simulink model "Active_Suspension_Control_Simulink_TEST"  (R2023b)
settings: Solver=FixedStepAuto  StartTime=0.0  StopTime=10  FixedStep=0.001  MaxStep=1e-3  RelTol=1e-3
values from neighbouring files (symbols this model uses):
  a = [1 20 3486.66666667 10555.5555556 168888.888889]    [Fuzzy_Workspace.mat]    (also in quarter_car_model.m = 0.8)
  b = [0 0 0.00333333333333 10555.6111112 168900.333335]    [Fuzzy_Workspace.mat]
  c_car = 1000    [Active_Suspension_Control.m]    (also in Fuzzy_Workspace.mat)
  k_car = 16000    [Active_Suspension_Control.m]    (also in Fuzzy_Workspace.mat)
  k_wheel = 190000    [Active_Suspension_Control.m]    (also in Fuzzy_Workspace.mat)
  m_car = 300    [Active_Suspension_Control.m]    (also in Fuzzy_Workspace.mat)
  m_wheel = 60    [Active_Suspension_Control.m]    (also in Fuzzy_Workspace.mat)
libraries: slpidlib x2, fuzblock x1, simulink x1
settings Model: Creator=hkurt  LastModifiedBy=hkurt
settings SolverCC: ZeroCrossControl=DisableAll  EnableFixedStepZeroCrossing=on

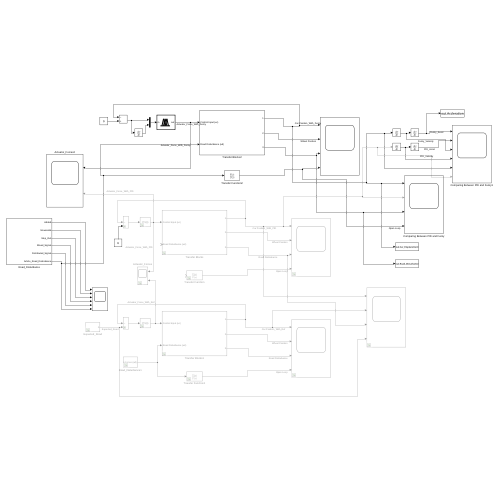
[thumbnail: Simulink's stored preview of the top-level diagram]
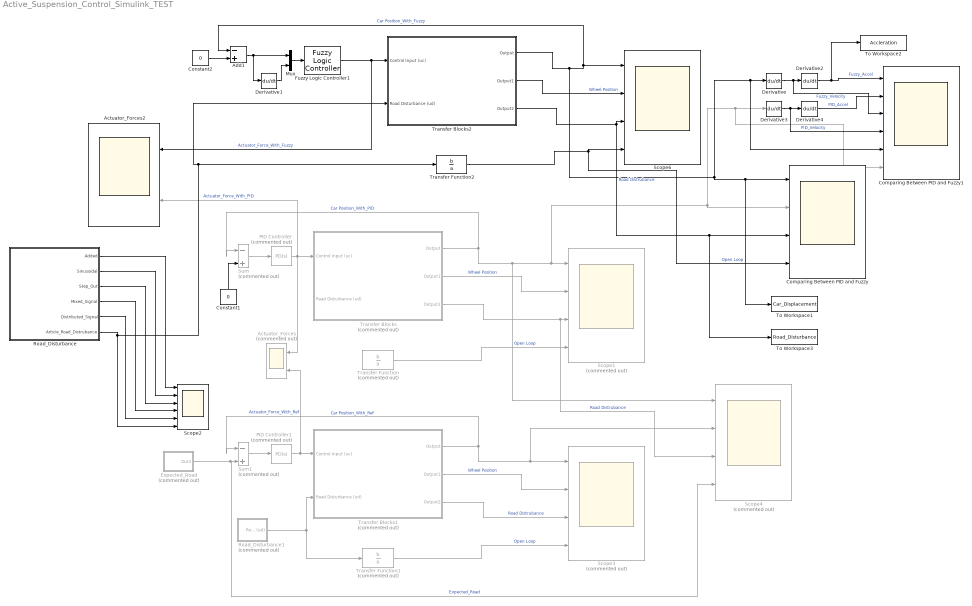
== system Active_Suspension_Control_Simulink_TEST ==
  Actuator_Forces : Scope  Commented=on  NumInputPorts=2
  Actuator_Forces2 : Scope  NumInputPorts=2
  Add1 : Sum  Inputs=-+
  Comparing Between PID and Fuzzy : Scope  NumInputPorts=4
  Comparing Between PID and Fuzzy1 : Scope  NumInputPorts=6
  Constant1 : Constant  Value=0
  Constant2 : Constant  Value=0
  Derivative{,1..4} (5 alike) : Derivative
  Expected_Road : Subsystem  Commented=on
  Fuzzy Logic Controller1 : fuzblock/Fuzzy Logic  Controller  FIS=my_fuzzy_8  OutputSampleNumber=101  DataType=double  FuzzifiedInputs=off  RuleFiringStrengths=off  RuleOutputs=off  AggregatedOutputs=off  SimulateUsing=Interpreted execution  OutOfRangeInputValueMessage=warning  NoRuleFiredMessage=warning  EmptyOutputFuzzySetMessage=warning
  Mux : Mux  Inputs=2
  PID Controller : slpidlib/PID Controller  Commented=on  Controller=PD  Form=Parallel  TimeDomain=Continuous-time  UseExternalTs=off  SampleTime=-1  IntegratorMethod=Forward Euler  FilterMethod=Forward Euler  ControllerParametersSource=internal  P=0.01  I=1000  UseKiTs=off  D=10000  N=100  UseFilter=on  TunerSelectOption=Transfer Function Based (PID Tuner App)  InitialConditionSource=internal  InitialConditionForIntegrator=0  InitialConditionForFilter=0  DifferentiatorICPrevScaledInput=0  ExternalReset=none  TrackingMode=off  Kt=1  LimitOutput=off  SatLimitsSource=internal  UpperSaturationLimit=2000  LowerSaturationLimit=-2000  LinearizeAsGain=on  AntiWindupMode=none  Kb=1  LimitIntegrator=off  UpperIntegratorSaturationLimit=inf  LowerIntegratorSaturationLimit=-inf  POutMin=[]  POutMax=[]  IOutMin=[]  IOutMax=[]  DOutMin=[]  DOutMax=[]  NOutMin=[]  NOutMax=[]  SumOutMin=[]  SumOutMax=[]  SaturationOutMin=[]  SaturationOutMax=[]  PParamMin=[]  PParamMax=[]  IParamMin=[]  IParamMax=[]  DParamMin=[]  DParamMax=[]  NParamMin=[]  NParamMax=[]  KbParamMin=[]  KbParamMax=[]  KtParamMin=[]  KtParamMax=[]  KbOutMin=[]  KbOutMax=[]  KtOutMin=[]  KtOutMax=[]  IntegratorOutMin=[]  IntegratorOutMax=[]  FilterOutMin=[]  FilterOutMax=[]  SumI1OutMin=[]  SumI1OutMax=[]  SumI2OutMin=[]  SumI2OutMax=[]  SumI3OutMin=[]  SumI3OutMax=[]  SumI4OutMin=[]  SumI4OutMax=[]  SumDOutMin=[]  SumDOutMax=[]  DifferentiatorOutMin=[]  DifferentiatorOutMax=[]  FilterDiffOutCoefMin=[]  FilterDiffOutCoefMax=[]  ReciprocalOutMin=[]  ReciprocalOutMax=[]  SumDenOutMin=[]  SumDenOutMax=[]  SumNumOutMin=[]  SumNumOutMax=[]  DivideOutMin=[]  DivideOutMax=[]  UdiffTsProdOutMin=[]  UdiffTsProdOutMax=[]  NTsProdOutMin=[]  NTsProdOutMax=[]  UintegralTsProdOutMin=[]  UintegralTsProdOutMax=[]  UngainTsProdOutMin=[]  UngainTsProdOutMax=[]  ClampingZeroOutDataTypeStr=Inherit: Inherit via back propagation  ClampingZeroOutMin=[]  ClampingZeroOutMax=[]  FilterDenConstantOutDataTypeStr=Inherit: Inherit via back propagation  FilterDenConstantOutMin=[]  FilterDenConstantOutMax=[]  PCopyOutDataTypeStr=Inherit: Inherit via back propagation  PCopyOutMin=[]  PCopyOutMax=[]  NCopyOutDataTypeStr=Inherit: Inherit via back propagation  NCopyOutMin=[]  NCopyOutMax=[]  IntegratorContinuousStateAttributes=''  IntegratorStateMustResolveToSignalObject=off  IntegratorRTWStateStorageClass=Auto  FilterContinuousStateAttributes=''  FilterStateMustResolveToSignalObject=off  FilterRTWStateStorageClass=Auto  ParallelPVariant=InternalParameters  IdealPVariant=Disabled  IVariant=Disabled  DVariant=InternalParameters  IntegratorVariant=Disabled  SatVariant=Disabled  AWVariant=Disabled  PCopyVariant=Disabled  TRVariant=Disabled  FdbkBlocksVariant=Forward  IdealPFdbkVariant=Disabled  SatFdbkVariant=Disabled  DerivativeFilterVariant=ContFilter  NVariant=InternalParameters  NCopyVariant=Disabled  FilterICVariant=InternalICsFilter  IntegratorICVariant=Disabled  ExternalResetVariant=Disabled  TRSumVariant=Passthrough  SumFdbkVariant=Disabled  SumVariant=Sum_PD  TsampFilterVariant=InternalTs  TsampNgainVariant=Passthrough  TsampIntegralVariant=Disabled_SignalSpec  ExternalSaturationOutDataTypeStr=Inherit: Same as second input
  PID Controller1 : slpidlib/PID Controller  Commented=on  Controller=PD  Form=Parallel  TimeDomain=Continuous-time  UseExternalTs=off  SampleTime=-1  IntegratorMethod=Forward Euler  FilterMethod=Forward Euler  ControllerParametersSource=internal  P=0.01  I=1000  UseKiTs=off  D=10000  N=100  UseFilter=on  TunerSelectOption=Transfer Function Based (PID Tuner App)  InitialConditionSource=internal  InitialConditionForIntegrator=0  InitialConditionForFilter=0  DifferentiatorICPrevScaledInput=0  ExternalReset=none  TrackingMode=off  Kt=1  LimitOutput=off  SatLimitsSource=internal  UpperSaturationLimit=2000  LowerSaturationLimit=-2000  LinearizeAsGain=on  AntiWindupMode=none  Kb=1  LimitIntegrator=off  UpperIntegratorSaturationLimit=inf  LowerIntegratorSaturationLimit=-inf  POutMin=[]  POutMax=[]  IOutMin=[]  IOutMax=[]  DOutMin=[]  DOutMax=[]  NOutMin=[]  NOutMax=[]  SumOutMin=[]  SumOutMax=[]  SaturationOutMin=[]  SaturationOutMax=[]  PParamMin=[]  PParamMax=[]  IParamMin=[]  IParamMax=[]  DParamMin=[]  DParamMax=[]  NParamMin=[]  NParamMax=[]  KbParamMin=[]  KbParamMax=[]  KtParamMin=[]  KtParamMax=[]  KbOutMin=[]  KbOutMax=[]  KtOutMin=[]  KtOutMax=[]  IntegratorOutMin=[]  IntegratorOutMax=[]  FilterOutMin=[]  FilterOutMax=[]  SumI1OutMin=[]  SumI1OutMax=[]  SumI2OutMin=[]  SumI2OutMax=[]  SumI3OutMin=[]  SumI3OutMax=[]  SumI4OutMin=[]  SumI4OutMax=[]  SumDOutMin=[]  SumDOutMax=[]  DifferentiatorOutMin=[]  DifferentiatorOutMax=[]  FilterDiffOutCoefMin=[]  FilterDiffOutCoefMax=[]  ReciprocalOutMin=[]  ReciprocalOutMax=[]  SumDenOutMin=[]  SumDenOutMax=[]  SumNumOutMin=[]  SumNumOutMax=[]  DivideOutMin=[]  DivideOutMax=[]  UdiffTsProdOutMin=[]  UdiffTsProdOutMax=[]  NTsProdOutMin=[]  NTsProdOutMax=[]  UintegralTsProdOutMin=[]  UintegralTsProdOutMax=[]  UngainTsProdOutMin=[]  UngainTsProdOutMax=[]  ClampingZeroOutDataTypeStr=Inherit: Inherit via back propagation  ClampingZeroOutMin=[]  ClampingZeroOutMax=[]  FilterDenConstantOutDataTypeStr=Inherit: Inherit via back propagation  FilterDenConstantOutMin=[]  FilterDenConstantOutMax=[]  PCopyOutDataTypeStr=Inherit: Inherit via back propagation  PCopyOutMin=[]  PCopyOutMax=[]  NCopyOutDataTypeStr=Inherit: Inherit via back propagation  NCopyOutMin=[]  NCopyOutMax=[]  IntegratorContinuousStateAttributes=''  IntegratorStateMustResolveToSignalObject=off  IntegratorRTWStateStorageClass=Auto  FilterContinuousStateAttributes=''  FilterStateMustResolveToSignalObject=off  FilterRTWStateStorageClass=Auto  ParallelPVariant=InternalParameters  IdealPVariant=Disabled  IVariant=Disabled  DVariant=InternalParameters  IntegratorVariant=Disabled  SatVariant=Disabled  AWVariant=Disabled  PCopyVariant=Disabled  TRVariant=Disabled  FdbkBlocksVariant=Forward  IdealPFdbkVariant=Disabled  SatFdbkVariant=Disabled  DerivativeFilterVariant=ContFilter  NVariant=InternalParameters  NCopyVariant=Disabled  FilterICVariant=InternalICsFilter  IntegratorICVariant=Disabled  ExternalResetVariant=Disabled  TRSumVariant=Passthrough  SumFdbkVariant=Disabled  SumVariant=Sum_PD  TsampFilterVariant=InternalTs  TsampNgainVariant=Passthrough  TsampIntegralVariant=Disabled_SignalSpec  ExternalSaturationOutDataTypeStr=Inherit: Same as second input
  Road_Disturbance : Subsystem
  Road_Disturbance1 : Subsystem  Commented=on
  Scope1 : Scope  Commented=on  NumInputPorts=4
  Scope2 : Scope  NumInputPorts=6
  Scope3 : Scope  Commented=on  NumInputPorts=4
  Scope4 : Scope  Commented=on  NumInputPorts=4
  Scope6 : Scope  NumInputPorts=4
  Sum : Sum  Commented=on  Inputs=|-+
  Sum1 : Sum  Commented=on  Inputs=|-+
  To Workspace1 : ToWorkspace  VariableName=Car_Displacement  SaveFormat=Timeseries  SampleTime=-1
  To Workspace2 : ToWorkspace  VariableName=Accleration  SaveFormat=Timeseries  SampleTime=-1
  To Workspace3 : ToWorkspace  VariableName=Road_Disturbance  SaveFormat=Timeseries  SampleTime=-1
  Transfer Blocks : Subsystem  Commented=on
  Transfer Blocks1 : Subsystem  Commented=on
  Transfer Blocks2 : Subsystem
  Transfer Function : TransferFcn  Commented=on  Numerator=b  Denominator=a
  Transfer Function1 : TransferFcn  Commented=on  Numerator=b  Denominator=a
  Transfer Function2 : TransferFcn  Numerator=b  Denominator=a
  wires:
  Transfer Blocks/2(Output1) -> Scope1/2  "Wheel Position"
  Transfer Blocks/3(Output2) -> Scope4/3, Scope1/3  "Road Distrubance"
  Transfer Blocks/1(Output) -> Sum/1, Scope4/1, Comparing Between PID and Fuzzy1/6, Derivative3/1, Comparing Between PID and Fuzzy/2, Scope1/1  "Car Position_With_PID"
  Transfer Function/1 -> Scope1/4  "Open Loop"
  Sum/1 -> PID Controller/1
  PID Controller/1 -> Actuator_Forces2/2, Actuator_Forces/1, Transfer Blocks/1(Control Input (uc))  "Actuator_Force_With_PID"
  Transfer Function1/1 -> Scope3/4  "Open Loop"
  Transfer Blocks1/3(Output2) -> Scope3/3  "Road Distrubance"
  Sum1/1 -> PID Controller1/1
  Transfer Blocks1/1(Output) -> Sum1/1, Scope4/2, Scope3/1  "Car Position_With_Ref"
  Road_Disturbance1/1(Road Disturbance (ud)) -> Transfer Blocks1/2(Road Disturbance (ud)), Transfer Function1/1
  PID Controller1/1 -> Actuator_Forces/2, Transfer Blocks1/1(Control Input (uc))  "Actuator_Force_With_Ref"
  Transfer Blocks1/2(Output1) -> Scope3/2  "Wheel Position"
  Expected_Road/1(Out1) -> Scope4/4, Sum1/2  "Expected_Road"
  Constant1/1 -> Sum/2
  Transfer Function2/1 -> Comparing Between PID and Fuzzy/4, Scope6/4  "Open Loop"
  Transfer Blocks2/3(Output2) -> To Workspace3/1, Comparing Between PID and Fuzzy/3, Scope6/3  "Road Distrubance"
  Transfer Blocks2/2(Output1) -> Scope6/2  "Wheel Position"
  Transfer Blocks2/1(Output) -> Comparing Between PID and Fuzzy1/5, Derivative/1, To Workspace1/1, Comparing Between PID and Fuzzy/1, Add1/1, Scope6/1  "Car Position_With_Fuzzy"
  Add1/1 -> Derivative1/1, Mux/1
  Mux/1 -> Fuzzy Logic Controller1/1
  Derivative1/1 -> Mux/2
  Constant2/1 -> Add1/2
  Fuzzy Logic Controller1/1 -> Transfer Blocks2/1(Control Input (uc)), Actuator_Forces2/1  "Actuator_Force_With_Fuzzy"
  Derivative/1 -> Comparing Between PID and Fuzzy1/3, Derivative2/1  "Fuzzy_Velocity"
  Derivative3/1 -> Comparing Between PID and Fuzzy1/4, Derivative4/1  "PID_Velocity"
  Derivative4/1 -> Comparing Between PID and Fuzzy1/2  "PID_Accel"
  Derivative2/1 -> To Workspace2/1, Comparing Between PID and Fuzzy1/1  "Fuzzy_Accel"
  Road_Disturbance/1(Added) -> Scope2/1
  Road_Disturbance/2(Sinusoidal) -> Scope2/2
  Road_Disturbance/3(Step_Out) -> Scope2/3
  Road_Disturbance/4(Mixed_Signal) -> Scope2/4
  Road_Disturbance/5(Distributed_Signal) -> Scope2/5
  Road_Disturbance/6(Article_Road_Distrubance) -> Scope2/6, Transfer Blocks2/2(Road Disturbance (ud)), Transfer Function2/1

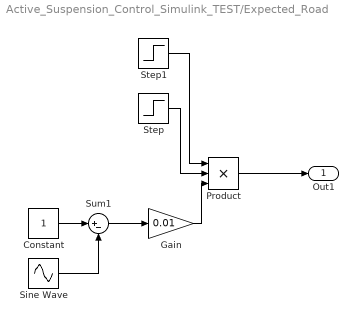
== system Active_Suspension_Control_Simulink_TEST/Expected_Road ==
  Constant : Constant
  Gain : Gain  Gain=0.01
  Product : Product  Inputs=3
  Sine Wave : Sin  Frequency=0.5*pi  Phase=pi/4  SampleTime=0
  Step : Step  Time=4.5  Before=1  After=0  SampleTime=0
  Step1 : Step  Time=0.5  SampleTime=0
  Sum1 : Sum  Inputs=|+-
  Out1 : Outport
  wires:
  Sine Wave/1 -> Sum1/2
  Sum1/1 -> Gain/1
  Gain/1 -> Product/3
  Step/1 -> Product/2
  Constant/1 -> Sum1/1
  Product/1 -> Out1/1
  Step1/1 -> Product/1

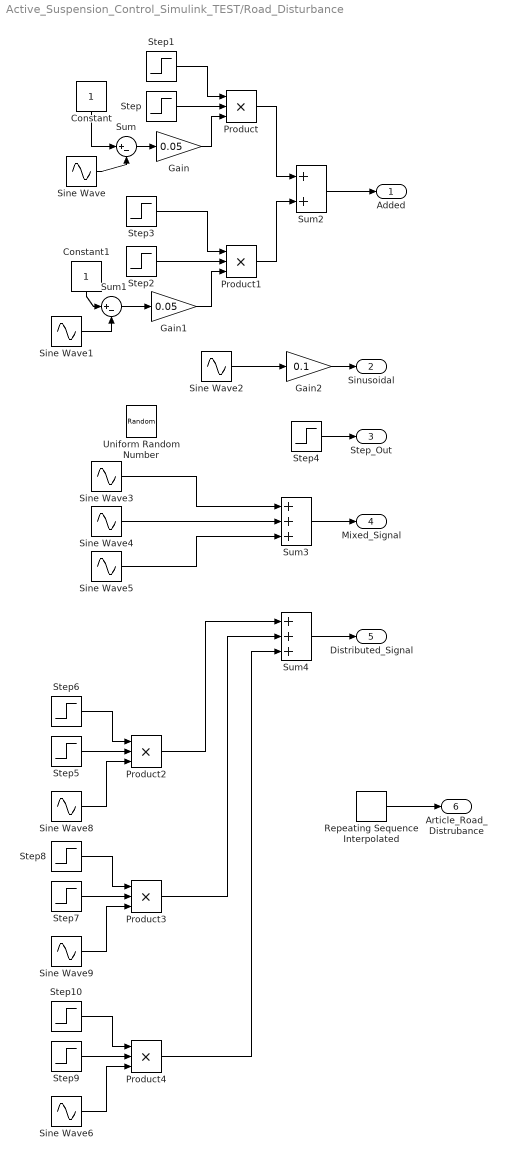
== system Active_Suspension_Control_Simulink_TEST/Road_Disturbance ==
  Constant : Constant
  Constant1 : Constant
  Gain : Gain  Gain=0.05
  Gain1 : Gain  Gain=0.05
  Gain2 : Gain  Gain=0.1
  Product{,1..4} (5 alike) : Product  Inputs=3
  Repeating Sequence Interpolated : simulink/Sources/Repeating Sequence Interpolated  OutValues=[0.0 -0.005 -0.012 -0.011 -0.015 0.012 0.009 0.028 0.024 0.020 0.026 0.028 0.020 -0.01 -0.012 -0.015 0.02 0.028 -0.018 0.02 0.015 0.012 -0.005 -0.013 0.007 0.0].'  TimeValues=[0 0.4 0.8 1.2 1.6 2.0 2.4 2.8 3.2 3.6 4.0 4.4 4.8 5.2 5.6 6.0 6.4 6.8 7.2 7.6 8.0 8.4 8.8 9.2 9.6 10.0].'  LookUpMeth=Interpolation-Use End Values  tsamp=0.01  OutMin=[]  OutMax=[]  OutDataTypeStr=double  OutputDataTypeScalingMode=double  OutDataType=fixdt(0,8)  OutScaling=2^-10
  Sine Wave : Sin  Frequency=2*pi  Phase=pi*3/2  SampleTime=0
  Sine Wave1 : Sin  Frequency=2*pi  Phase=pi*3/2  SampleTime=0
  Sine Wave2 : Sin  Frequency=2*pi  Phase=pi  SampleTime=0
  Sine Wave3 : Sin  Amplitude=0.01  Frequency=15*pi  SampleTime=0
  Sine Wave4 : Sin  Amplitude=0.02  Frequency=10*pi  Phase=pi/2  SampleTime=0
  Sine Wave5 : Sin  Amplitude=0.03  Frequency=pi  SampleTime=0
  Sine Wave6 : Sin  Amplitude=0.08  Frequency=pi  Phase=pi*3/2  SampleTime=0
  Sine Wave8 : Sin  Amplitude=0.1  Frequency=pi  Phase=pi*3/2  SampleTime=0
  Sine Wave9 : Sin  Amplitude=0.05  Frequency=pi  Phase=pi*3/2  SampleTime=0
  Step : Step  Time=1.5  Before=1  After=0  SampleTime=0
  Step1 : Step  Time=0.5  SampleTime=0
  Step10 : Step  Time=8.5  SampleTime=0
  Step2 : Step  Time=3.5  Before=1  After=0  SampleTime=0
  Step3 : Step  Time=2.5  SampleTime=0
  Step4 : Step  Time=2  After=0.015  SampleTime=0
  Step5 : Step  Time=1.5  Before=1  After=0  SampleTime=0
  Step6 : Step  Time=0.5  SampleTime=0
  Step7 : Step  Time=5.5  Before=1  After=0  SampleTime=0
  Step8 : Step  Time=4.5  SampleTime=0
  Step9 : Step  Time=9.5  Before=1  After=0  SampleTime=0
  Sum : Sum  Inputs=|+-
  Sum1 : Sum  Inputs=|+-
  Sum2 : Sum
  Sum3 : Sum  Inputs=+++
  Sum4 : Sum  Inputs=+++
  Uniform Random Number : UniformRandomNumber  Minimum=-0.05  Maximum=0.05  SampleTime=0.1
  Added : Outport
  Sinusoidal : Outport  Port=2
  Step_Out : Outport  Port=3
  Mixed_Signal : Outport  Port=4
  Distributed_Signal : Outport  Port=5
  Article_Road_Distrubance : Outport  Port=6
  wires:
  Constant/1 -> Sum/1
  Step/1 -> Product/2
  Sum/1 -> Gain/1
  Gain/1 -> Product/3
  Sine Wave/1 -> Sum/2
  Step1/1 -> Product/1
  Gain1/1 -> Product1/3
  Step2/1 -> Product1/2
  Step3/1 -> Product1/1
  Product1/1 -> Sum2/2
  Product/1 -> Sum2/1
  Constant1/1 -> Sum1/1
  Sine Wave1/1 -> Sum1/2
  Sum1/1 -> Gain1/1
  Sine Wave2/1 -> Gain2/1
  Sum2/1 -> Added/1
  Gain2/1 -> Sinusoidal/1
  Step4/1 -> Step_Out/1
  Sum3/1 -> Mixed_Signal/1
  Sine Wave3/1 -> Sum3/1
  Sine Wave4/1 -> Sum3/2
  Sine Wave5/1 -> Sum3/3
  Step6/1 -> Product2/1
  Product2/1 -> Sum4/1
  Step5/1 -> Product2/2
  Sine Wave8/1 -> Product2/3
  Sum4/1 -> Distributed_Signal/1
  Step8/1 -> Product3/1
  Step7/1 -> Product3/2
  Sine Wave9/1 -> Product3/3
  Product3/1 -> Sum4/2
  Step10/1 -> Product4/1
  Step9/1 -> Product4/2
  Sine Wave6/1 -> Product4/3
  Product4/1 -> Sum4/3
  Repeating Sequence Interpolated/1 -> Article_Road_Distrubance/1

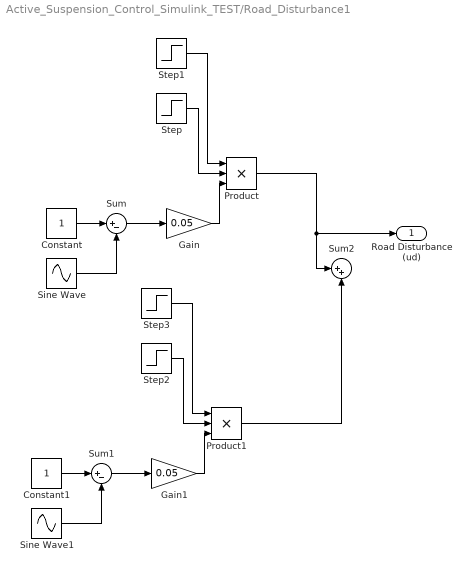
== system Active_Suspension_Control_Simulink_TEST/Road_Disturbance1 ==
  Constant : Constant
  Constant1 : Constant
  Gain : Gain  Gain=0.05
  Gain1 : Gain  Gain=0.05
  Product : Product  Inputs=3
  Product1 : Product  Inputs=3
  Sine Wave : Sin  Frequency=2*pi  Phase=pi*3/2  SampleTime=0
  Sine Wave1 : Sin  Frequency=2*pi  Phase=pi*3/2  SampleTime=0
  Step : Step  Time=1.5  Before=1  After=0  SampleTime=0
  Step1 : Step  Time=0.5  SampleTime=0
  Step2 : Step  Time=3.5  Before=1  After=0  SampleTime=0
  Step3 : Step  Time=2.5  SampleTime=0
  Sum : Sum  Inputs=|+-
  Sum1 : Sum  Inputs=|+-
  Sum2 : Sum  Inputs=|++
  Road Disturbance (ud) : Outport
  wires:
  Constant/1 -> Sum/1
  Step/1 -> Product/2
  Sum/1 -> Gain/1
  Gain/1 -> Product/3
  Sine Wave/1 -> Sum/2
  Step1/1 -> Product/1
  Sum1/1 -> Gain1/1
  Constant1/1 -> Sum1/1
  Gain1/1 -> Product1/3
  Sine Wave1/1 -> Sum1/2
  Step2/1 -> Product1/2
  Step3/1 -> Product1/1
  Product/1 -> Sum2/1, Road Disturbance (ud)/1
  Product1/1 -> Sum2/2

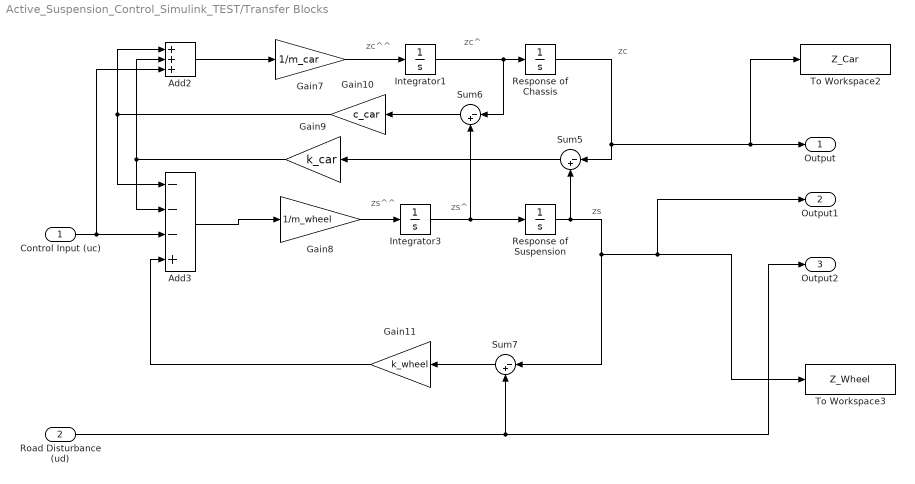
== system Active_Suspension_Control_Simulink_TEST/Transfer Blocks ==
  note: zs
  note: zc^^
  note: zc
  note: zc^
  note: zs^^
  note: zs^
  Control Input (uc) : Inport
  Road Disturbance (ud) : Inport  Port=2
  Add2 : Sum  Inputs=+++
  Add3 : Sum  Inputs=---+
  Gain10 : Gain  Gain=c_car
  Gain11 : Gain  Gain=k_wheel
  Gain7 : Gain  Gain=1/m_car
  Gain8 : Gain  Gain=1/m_wheel
  Gain9 : Gain  Gain=k_car
  Integrator1 : Integrator
  Integrator3 : Integrator
  Response of Chassis : Integrator
  Response of Suspension : Integrator
  Sum5 : Sum  Inputs=|-+
  Sum6 : Sum  Inputs=|-+
  Sum7 : Sum  Inputs=|-+
  To Workspace2 : ToWorkspace  VariableName=Z_Car  SaveFormat=Timeseries  SampleTime=-1
  To Workspace3 : ToWorkspace  VariableName=Z_Wheel  SaveFormat=Timeseries  SampleTime=-1
  Output : Outport
  Output1 : Outport  Port=2
  Output2 : Outport  Port=3
  wires:
  Gain11/1 -> Add3/4
  Sum5/1 -> Gain9/1
  Add3/1 -> Gain8/1
  Response of Suspension/1 -> Sum5/2, Sum7/1, Output1/1, To Workspace3/1
  Sum7/1 -> Gain11/1
  Integrator1/1 -> Sum6/1, Response of Chassis/1
  Gain8/1 -> Integrator3/1
  Gain9/1 -> Add3/2, Add2/2
  Sum6/1 -> Gain10/1
  Response of Chassis/1 -> Sum5/1, Output/1, To Workspace2/1
  Gain7/1 -> Integrator1/1
  Road Disturbance (ud)/1 -> Sum7/2, Output2/1
  Integrator3/1 -> Sum6/2, Response of Suspension/1
  Add2/1 -> Gain7/1
  Gain10/1 -> Add3/1, Add2/1
  Control Input (uc)/1 -> Add2/3, Add3/3

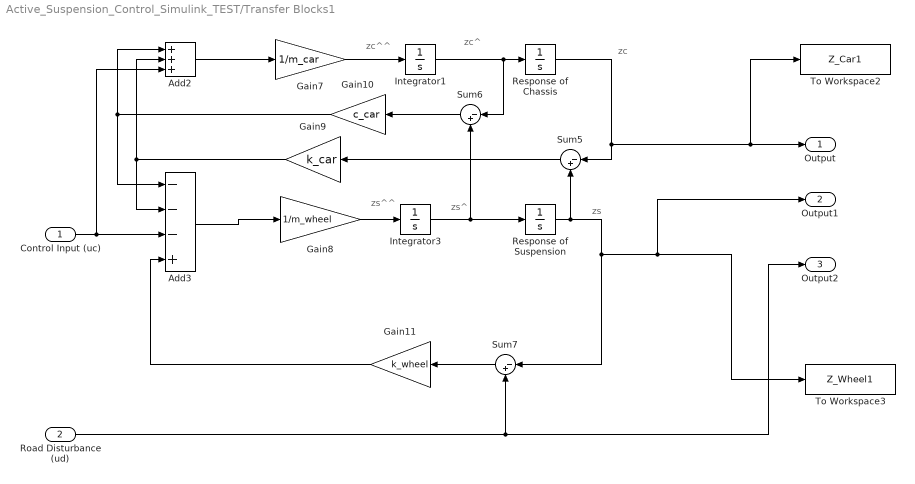
== system Active_Suspension_Control_Simulink_TEST/Transfer Blocks1 ==
  note: zs
  note: zc^^
  note: zc
  note: zc^
  note: zs^^
  note: zs^
  Control Input (uc) : Inport
  Road Disturbance (ud) : Inport  Port=2
  Add2 : Sum  Inputs=+++
  Add3 : Sum  Inputs=---+
  Gain10 : Gain  Gain=c_car
  Gain11 : Gain  Gain=k_wheel
  Gain7 : Gain  Gain=1/m_car
  Gain8 : Gain  Gain=1/m_wheel
  Gain9 : Gain  Gain=k_car
  Integrator1 : Integrator
  Integrator3 : Integrator
  Response of Chassis : Integrator
  Response of Suspension : Integrator
  Sum5 : Sum  Inputs=|-+
  Sum6 : Sum  Inputs=|-+
  Sum7 : Sum  Inputs=|-+
  To Workspace2 : ToWorkspace  VariableName=Z_Car1  SaveFormat=Timeseries  SampleTime=-1
  To Workspace3 : ToWorkspace  VariableName=Z_Wheel1  SaveFormat=Timeseries  SampleTime=-1
  Output : Outport
  Output1 : Outport  Port=2
  Output2 : Outport  Port=3
  wires:
  Gain11/1 -> Add3/4
  Sum5/1 -> Gain9/1
  Add3/1 -> Gain8/1
  Response of Suspension/1 -> Sum5/2, Sum7/1, Output1/1, To Workspace3/1
  Sum7/1 -> Gain11/1
  Integrator1/1 -> Sum6/1, Response of Chassis/1
  Gain8/1 -> Integrator3/1
  Gain9/1 -> Add3/2, Add2/2
  Sum6/1 -> Gain10/1
  Response of Chassis/1 -> Sum5/1, Output/1, To Workspace2/1
  Gain7/1 -> Integrator1/1
  Road Disturbance (ud)/1 -> Sum7/2, Output2/1
  Integrator3/1 -> Sum6/2, Response of Suspension/1
  Add2/1 -> Gain7/1
  Gain10/1 -> Add3/1, Add2/1
  Control Input (uc)/1 -> Add2/3, Add3/3

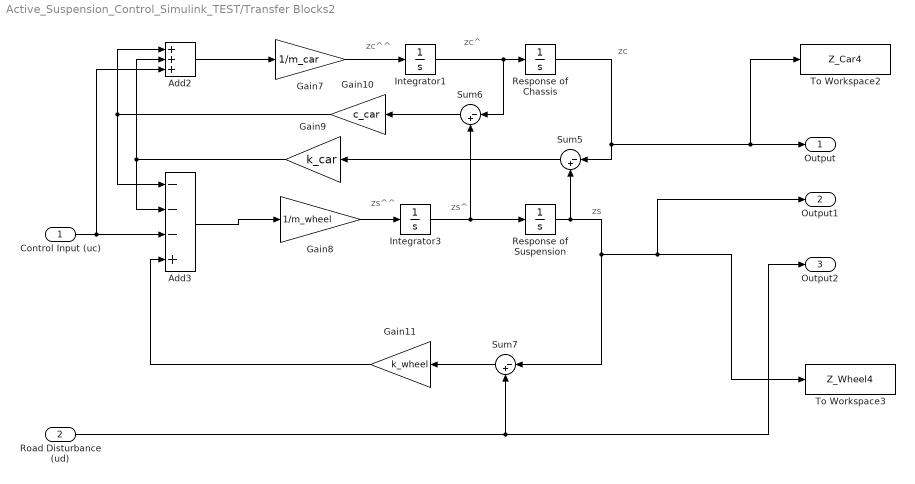
== system Active_Suspension_Control_Simulink_TEST/Transfer Blocks2 ==
  note: zs
  note: zc^^
  note: zc
  note: zc^
  note: zs^^
  note: zs^
  Control Input (uc) : Inport
  Road Disturbance (ud) : Inport  Port=2
  Add2 : Sum  Inputs=+++
  Add3 : Sum  Inputs=---+
  Gain10 : Gain  Gain=c_car
  Gain11 : Gain  Gain=k_wheel
  Gain7 : Gain  Gain=1/m_car
  Gain8 : Gain  Gain=1/m_wheel
  Gain9 : Gain  Gain=k_car
  Integrator1 : Integrator
  Integrator3 : Integrator
  Response of Chassis : Integrator
  Response of Suspension : Integrator
  Sum5 : Sum  Inputs=|-+
  Sum6 : Sum  Inputs=|-+
  Sum7 : Sum  Inputs=|-+
  To Workspace2 : ToWorkspace  VariableName=Z_Car4  SaveFormat=Timeseries  SampleTime=-1
  To Workspace3 : ToWorkspace  VariableName=Z_Wheel4  SaveFormat=Timeseries  SampleTime=-1
  Output : Outport
  Output1 : Outport  Port=2
  Output2 : Outport  Port=3
  wires:
  Gain11/1 -> Add3/4
  Sum5/1 -> Gain9/1
  Add3/1 -> Gain8/1
  Response of Suspension/1 -> Sum5/2, Sum7/1, Output1/1, To Workspace3/1
  Sum7/1 -> Gain11/1
  Integrator1/1 -> Sum6/1, Response of Chassis/1
  Gain8/1 -> Integrator3/1
  Gain9/1 -> Add3/2, Add2/2
  Sum6/1 -> Gain10/1
  Response of Chassis/1 -> Sum5/1, Output/1, To Workspace2/1
  Gain7/1 -> Integrator1/1
  Road Disturbance (ud)/1 -> Sum7/2, Output2/1
  Integrator3/1 -> Sum6/2, Response of Suspension/1
  Add2/1 -> Gain7/1
  Gain10/1 -> Add3/1, Add2/1
  Control Input (uc)/1 -> Add2/3, Add3/3
